simulink model "impdamp_ex"  (R2022b)
settings: Solver=ode45  StartTime=0.0  StopTime=10.0  RelTol=1e-3  EnableMultiTasking=on
InitFcn:
  | % Parameters
  | k = 4.9;
  | b = 1.8;
  | m = 1;
libraries: SignalEditorBlockLib x1
settings Model: Creator=nicholas  LastModifiedBy=bensweet
settings SolverCC: AlgebraicLoopSolver=TrustRegion  MaxZcPerStep=1
settings DataIOCC: LimitDataPoints=on  SaveFormat=Array  ReturnWorkspaceOutputs=off  SignalLoggingName=sigsOut
settings OptimizationCC: ExpressionDepthLimit=2147483647  InitFltsAndDblsToZero=on  LifeSpan=inf
settings DebuggingCC: UnconnectedInputMsg=warning  UnconnectedOutputMsg=warning  UnconnectedLineMsg=warning  PregeneratedLibrarySubsystemCodeDiagnostic=none  SFMachineParentedDataDiag=warning
settings HardwareCC: ProdBitPerPointer=32  ProdBitPerSizeT=32  ProdBitPerPtrDiffT=32  ProdLargestAtomicFloat=None  ProdIntDivRoundTo=Undefined  ProdEndianess=Unspecified  ProdWordSize=32  ProdHWDeviceType=32-bit Generic  TargetUnknown=on
settings ModelReferenceCC: EnableRefExpFcnMdlSchedulingChecks=on  PropagateSignalLabelsOutOfModel=off
settings SFSimCC: SimUseLocalCustomCode=off
settings RTWCC: RTWUseLocalCustomCode=off  DLArmComputeVersion=19.05
settings CodeAppCC: StateflowObjectComments=on
settings GRTTargetCC: TargetFcnLib=ansi_tfl_tmw.mat  TargetLangStandard=C89/C90 (ANSI)  CombineOutputUpdateFcns=off  GRTInterface=on
settings ConfigComp: CovMetricSettings=dw  CovSaveCumulativeToWorkspaceVar=on  CovSaveSingleToWorkspaceVar=on  CovExternalEMLEnable=off  CovSFcnEnable=off

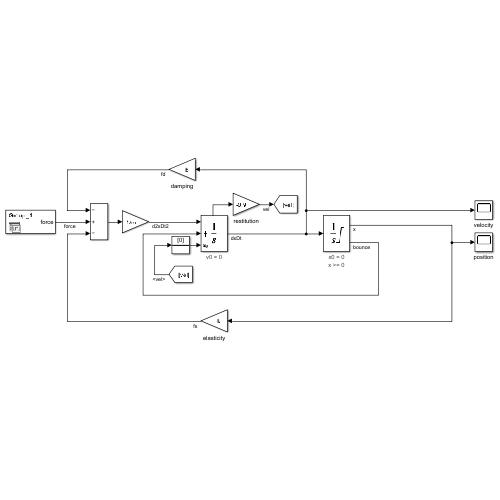
[thumbnail: Simulink's stored preview of the top-level diagram]
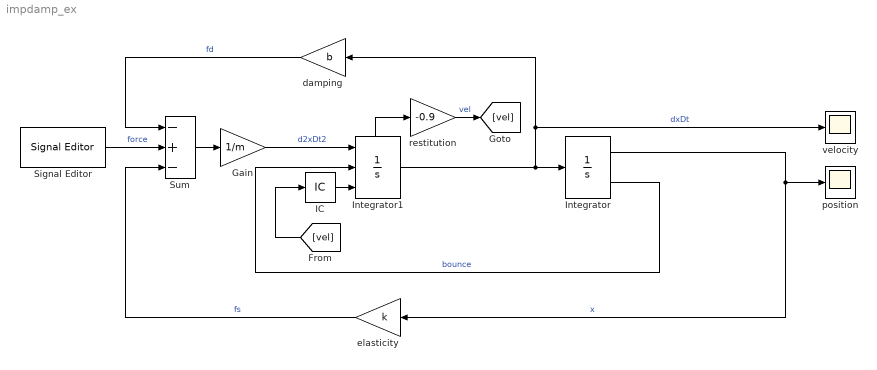
== system impdamp_ex ==
  Gain : Gain  Gain=1/m  SaturateOnIntegerOverflow=on  OutDataTypeStr=Inherit: Same as input  ParamDataTypeStr=Inherit: Same as input
  IC : InitialCondition  Value=0
  Integrator : Integrator  LimitOutput=on  LowerSaturationLimit=0  ShowSaturationPort=on
      settings: AttributesFormatString=x0 = %<InitialCondition>\nx >= %<LowerSaturationLimit>\n
  Integrator1 : Integrator  ExternalReset=falling  InitialConditionSource=external  ShowStatePort=on
      settings: AttributesFormatString=v0 = %<InitialCondition>\n
  Signal Editor : SignalEditorBlockLib/Signal Editor  FileName=impact_damper_force_dataset.mat  ActiveScenario=Group_1  ActiveSignal=force  IsBus=off  OutputBusObjectStr=Bus: BusObject  SampleTime=0  ZeroCross=off  OutputAfterFinalValue=Extrapolation  Unit=inherit  PreserveSignalName=on
  Sum : Sum  Inputs=-+-  SaturateOnIntegerOverflow=on
  damping : Gain  Gain=b  SaturateOnIntegerOverflow=on  OutDataTypeStr=Inherit: Same as input  ParamDataTypeStr=Inherit: Same as input
  elasticity : Gain  Gain=k  SaturateOnIntegerOverflow=on  OutDataTypeStr=Inherit: Same as input  ParamDataTypeStr=Inherit: Same as input
  position : Scope
  restitution : Gain  Gain=-0.9  SaturateOnIntegerOverflow=on  OutDataTypeStr=Inherit: Same as input  ParamDataTypeStr=Inherit: Same as input
  velocity : Scope
  wires:
  Integrator1/1 -> Integrator/1, velocity/1, damping/1  "dxDt"
  Integrator/1 -> elasticity/1, position/1  "x"
  elasticity/1 -> Sum/3  "fs"
  Sum/1 -> Gain/1
  Gain/1 -> Integrator1/1  "d2xDt2"
  Integrator1/State -> restitution/1
  IC/1 -> Integrator1/3
  Integrator/2 -> Integrator1/2  "bounce"
  Signal Editor/1 -> Sum/2  "force"
  damping/1 -> Sum/1  "fd"
  restitution/1 -> [vel]  "vel"
  [vel] -> IC/1
